simulink model "motoraiSIL"  (R2018b)
settings: Solver=FixedStepAuto  StartTime=0.0  StopTime=inf  FixedStep=SAMPLE_TIME  RelTol=1e-3  EnableMultiTasking=on
InitFcn:
  | UserSettings
values from neighbouring files (symbols this model uses):
  DATA_SAMPLING_FREQUENCY = 500    [UserSettings.m]
  ESTIMATION_SAMPLES = 50    [UserSettings.m]
  I = 0.0021    [LQG_control_design.m]    (also in LQR_control_design.m; UserSettings.m = 7.2e-08)
  i_max = 20    [LQG_control_design.m]    (also in LQR_control_design.m; UserSettings.m = 1)
  motorParameters = Parameters()    [UserSettings.m]
  omega_max = 20    [LQG_control_design.m]    (also in LQR_control_design.m; UserSettings.m)
  parameter_ranges = motorParameters.getNormRanges()    [UserSettings.m]
  SAMPLE_TIME = 1e-5    (= 1e-05)    [UserSettings.m]
  V_ACT = 1000    [UserSettings.m]
  v_max = 10    [LQG_control_design.m]    (also in LQR_control_design.m; UserSettings.m)
undefined symbols (not defined in the file or in its folder): myLQR, myREF
libraries: neural x230, fl_lib x5, nesl_utility x5, elec_lib x3, dspbuff3 x2, dspswit3 x1
(part 8 of 11)

== system motoraiSIL/Parameter Estimation & LQR /Function Fitting Neural Network1/Layer 2/Delays 1 ==
  "p{2}" : Inport  PortDimensions=166
      mask Display: e = 0.06;c1 = [120 230 180]/255;c2 = ([120 230 180]+0)/(256+128);c3 = ([120 230 180]+128)/(256+128);patch([0 1 1 0],[0 0 1 1],c1);patch([0 1 1 1-e 1-e 0+e],[0 0 1 1-e 0+e 0+e],c2);patch([0 0 1 1-e 0+e 0+e],[0 1 1 1-e 1-e 0+e],c3);plot([0 1 1 0 0],[0 0 1 1 0]);
  mux : Mux  Inputs=1
      mask Display: e = 0.06;c1 = [120 150 230]/255;c2 = ([120 150 230]+0)/383;c3 = ([120 150 230]+128)/383;patch([0 1 1 0],[0 0 1 1],c1);patch([0 1 1 1-e 1-e 0+e],[0 0 1 1-e 0+e 0+e],c2);patch([0 0 1 1-e 0+e 0+e],[0 1 1 1-e 1-e 0+e],c3);plot([0 1 1 0 0],[0 0 1 1 0]);disp('Mux')
  "pd{2,1}" : Outport
      mask Display: e = 0.06;c1 = [120 230 180]/255;c2 = ([120 230 180]+0)/(256+128);c3 = ([120 230 180]+128)/(256+128);patch([0 1 1 0],[0 0 1 1],c1);patch([0 1 1 1-e 1-e 0+e],[0 0 1 1-e 0+e 0+e],c2);patch([0 0 1 1-e 0+e 0+e],[0 1 1 1-e 1-e 0+e],c3);plot([0 1 1 0 0],[0 0 1 1 0]);
  wires:
  "p{2}"/1 -> mux/1
  mux/1 -> "pd{2,1}"/1
